simulink model "lqr_period_afbs_simu"  (R2015a)
settings: Solver=ode23  SolverMode=SingleTasking  StartTime=0.0  StopTime=simu.time  RelTol=1e-3
values from neighbouring files (symbols this model uses):
  A = importdata(filename,delimiterIn,headerlinesIn)    [analysis_pi_from_log.m]    (also in lqr_period_afbs.m = plant.model_ss.a; lqr_period_ideal_m.m = plant.model_ss.a; plot_pi_from_log.m)
  B = plant.model_ss.b    [lqr_period_afbs.m]    (also in lqr_period_ideal_m.m)
  C = plant.model_ss.c    [lqr_period_afbs.m]    (also in lqr_period_ideal_m.m)
undefined symbols (not defined in the file): afbs_parameters
libraries: simulink x1
settings Model: CovSFcnEnable=off  ExtModeTrigMode=oneshot  ExtModeArmWhenConnect=off  Creator=The MathWorks Inc.  LastModifiedBy=Xiaotian
settings DataIOCC: LimitDataPoints=off  SaveOutput=off  SignalLogging=off  DSMLogging=off  SaveTime=off  SignalLoggingName=sigsOut
settings OptimizationCC: BooleanDataType=off  ExpressionDepthLimit=2147483647  InitFltsAndDblsToZero=on
settings DebuggingCC: SaveWithParameterizedLinksMsg=none  UnderspecifiedInitializationDetection=Classic  MergeDetectMultiDrivingBlocksExec=none  SignalResolutionControl=TryResolveAllWithWarning  MultiTaskDSMMsg=warning  MultiTaskCondExecSysMsg=none  IntegerOverflowMsg=none  FcnCallInpInsideContextMsg=UseLocalSettings  StateNameClashWarn=warning  IntegerSaturationMsg=none
settings HardwareCC: TargetUnknown=on
settings GRTTargetCC: TargetFcnLib=ansi_tfl_tmw.mat  CombineOutputUpdateFcns=off  GRTInterface=on

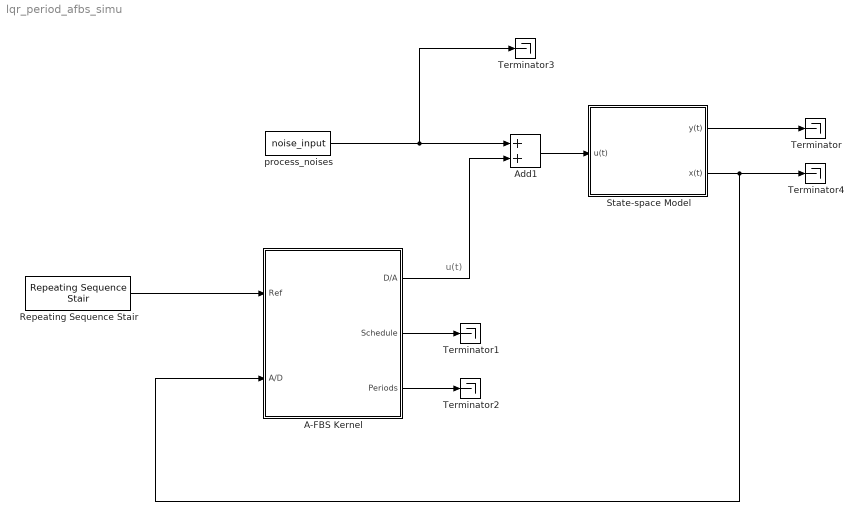
== system lqr_period_afbs_simu ==
  note: u(t)
  A-FBS Kernel : Subsystem  mask{para=afbs_parameters}
      mask prompts: para "A-FBS Parameters"
  Add1 : Sum
  Repeating Sequence Stair : simulink/Sources/Repeating Sequence Stair  OutValues=ref_sequence'  tsamp=ref_sampling_time  OutMin=[]  OutMax=[]  OutDataTypeStr=double  OutputDataTypeScalingMode=double  OutDataType=fixdt(0,8)  ConRadixGroup=Best Precision: Vector-wise  OutScaling=2^-12
  State-space Model : Subsystem  mask(State-space){A=A, B=B, C=C}
      mask help:
      | A state-space block using raw Simulink elements.
      | Internal states are exposed to use.
  Terminator{,1..4} (5 alike) : Terminator
  process_noises : FromWorkspace  VariableName=noise_input  SampleTime=0
  wires:
  A-FBS Kernel/1(D/A) -> Add1/2
  Add1/1 -> State-space Model/1(u(t))
  Repeating Sequence Stair/1 -> A-FBS Kernel/1(Ref)
  process_noises/1 -> Terminator3/1, Add1/1
  State-space Model/2(x(t)) -> Terminator4/1, A-FBS Kernel/2(A/D)
  State-space Model/1(y(t)) -> Terminator/1
  A-FBS Kernel/2(Schedule) -> Terminator1/1
  A-FBS Kernel/3(Periods) -> Terminator2/1

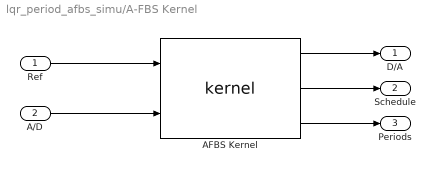
== system lqr_period_afbs_simu/A-FBS Kernel ==
  Ref : Inport
  A/D : Inport  Port=2
  AFBS Kernel : S-Function  FunctionName=kernel  Parameters=para
  D/A : Outport
  Schedule : Outport  Port=2
  Periods : Outport  Port=3
  wires:
  Ref/1 -> AFBS Kernel/1
  A/D/1 -> AFBS Kernel/2
  AFBS Kernel/2 -> Schedule/1
  AFBS Kernel/1 -> D/A/1
  AFBS Kernel/3 -> Periods/1

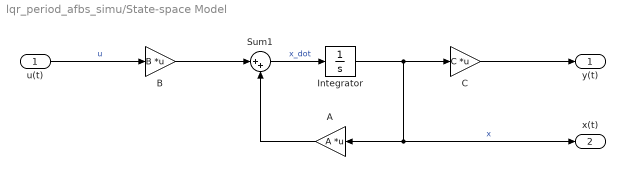
== system lqr_period_afbs_simu/State-space Model ==
  u(t) : Inport
  A : Gain  Gain=A  Multiplication=Matrix(K*u)
  B : Gain  Gain=B  Multiplication=Matrix(K*u)
  C : Gain  Gain=C  Multiplication=Matrix(K*u)
  Integrator : Integrator
  Sum1 : Sum  Inputs=|++
  y(t) : Outport
  x(t) : Outport  Port=2
  wires:
  u(t)/1 -> B/1  "u"
  B/1 -> Sum1/1
  A/1 -> Sum1/2
  Sum1/1 -> Integrator/1  "x_dot"
  Integrator/1 -> A/1, x(t)/1, C/1  "x"
  C/1 -> y(t)/1
